simulink model "dc_motor_starter_design_v4"  (R2025a)
settings: Solver=VariableStepAuto  StartTime=0.0  StopTime=8  RelTol=1e-3
libraries: spsDiodeLib x8, spsCurrentMeasurementLib x6, spsMosfetLib x5, simulink x4, spsMeanLib x4, spsSeriesRLCBranchLib x4, spsVoltageMeasurementLib x3, spsDCVoltageSourceLib x2, eePwmGenerator x2, spsACVoltageSourceLib x1, spsDCMachineLib x1, spsFirstOrderFilterLib x1
settings Model: Creator=Lenovo  LastModifiedBy=kaand

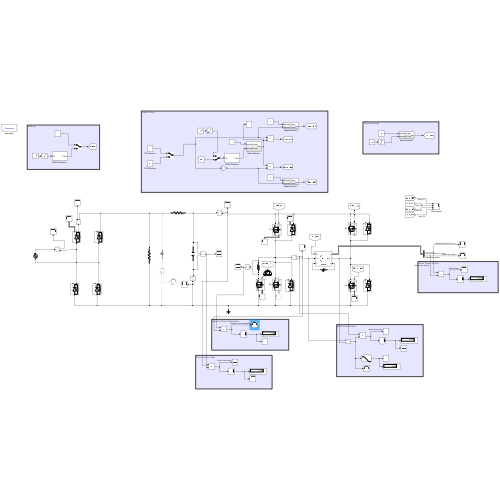
[thumbnail: Simulink's stored preview of the top-level diagram]
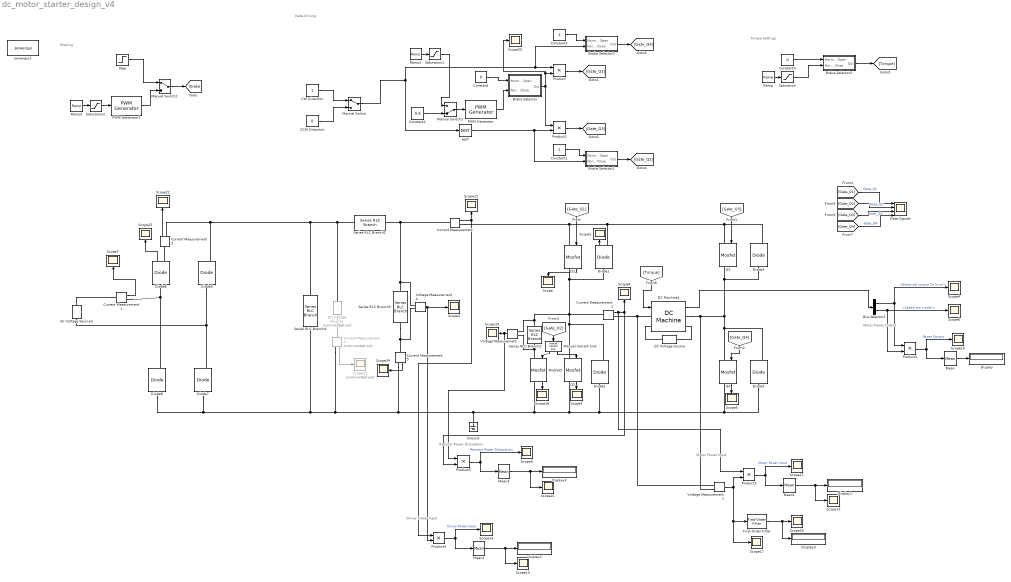
== system dc_motor_starter_design_v4 ==
  note: Torque Settings
  note: Gate Driving
  note: Resistor Power Dissipation
  note: Motor Power Input
  note: Motor Power Output
  note: Driver Power Input
  note: Braking
  AC Voltage Source3 : spsACVoltageSourceLib/AC Voltage Source  Amplitude=230  Phase=0  Frequency=50  SampleTime=0  Measurements=None  BusType=swing  Pref=10e3  Qref=0  Qmin=-inf  Qmax=+inf
  Brake Selector : Subsystem
  Brake Selector1 : Subsystem
  Brake Selector2 : Subsystem
  Brake Selector3 : Subsystem
  Bus Selector1 : BusSelector  OutputSignals=Electrical torque Te (n m),Speed wm (rad/s)
  CCW Direction : Constant  Value=0
  CW Direction : Constant
  Constant : Constant  Value=0
  Constant1 : Constant
  Constant2 : Constant  Value=0.6
  Constant3 : Constant
  Constant4 : Constant  Value=0
  Current Measurement{,1..3,5} (5 alike) : spsCurrentMeasurementLib/Current Measurement  PhasorSimulation=off  OutputType=Complex  PSBequivalent=0
  Current Measurement4 : spsCurrentMeasurementLib/Current Measurement  Commented=on  PhasorSimulation=off  OutputType=Complex  PSBequivalent=0
  DC Machine1 : spsDCMachineLib/DC Machine  PresetModel=No  MechanicalLoad=Torque TL  FieldType=Wound  ShowDetailedParameters=on  MeasurementBus=off  RLa="[ 0.8  0.0125]"  RLf="[ 210  23]"  Laf=1.8  MachineConstant=Torque constant (N.m/A)  Ke=1.8  Kt=1.8  J=1  Bm=0  Tf=0  w0=1  Ifinit=1.04761904756944  TsPowergui=0  TsBlock=-1
  DC Voltage Source : spsDCVoltageSourceLib/DC Voltage Source  Amplitude=220  Measurements=None
  DC Voltage Source1 : spsDCVoltageSourceLib/DC Voltage Source  Commented=on  Amplitude=200  Measurements=None
  Diode{1..8} (8 alike) : spsDiodeLib/Diode  Ron=0.036  Lon=0  Vf=1.1  IC=0  UseSnubber=0  Rs=500  Cs=250e-9  Measurements=on
  Display{,1..4} (5 alike) : Display
  First-Order Filter : spsFirstOrderFilterLib/First-Order Filter  FilterType=Lowpass  Tc=800e-6  Ts=0  Initialize=off  Vac_Init=[0, 0, 60]  Vdc_Init=0  PlotResponse=off  FreqRange="[0,  200,  1]"
  Gate Signals : Scope  NumInputPorts=4
      settings: ActiveDisplayYMinimum=-0.0065041846728933761  ActiveDisplayYMaximum=1.2434958153271063  DataLoggingVariableName=ScopeData21
  Ground : spsGroundLib/Ground  LConnTagsString=a
  Manual Variant Sink : simulink/Signal Routing/Manual Variant Sink  NumChoices=2  LabelModeActiveChoice=V_1
  Manual Switch : ManualSwitch
  Manual Switch1 : ManualSwitch  CurrentSetting=0
  Manual Switch2 : ManualSwitch
  Mean{,1..3} (4 alike) : spsMeanLib/Mean  Freq=50  Vinit=0  Ts=0
  Mosfet5 : spsMosfetLib/Mosfet  Ron=0.078  Lon=0  Rd=0.01  Vfd=0.7  IC=0  Rs=1e5  Cs=inf  Measurements=on
  NOT : Logic  Operator=NOT  IconShape=distinctive  AllPortsSameDT=off  OutDataTypeStr=boolean
  PWM Generator : eePwmGenerator/PWM Generator  CarrCount=Up  Tper=1/20e3  Tdelay=0  Ts=5e-6
  PWM Generator1 : eePwmGenerator/PWM Generator  CarrCount=Up  Tper=1/20e3  Tdelay=0  Ts=5e-6
  Product{,1..5} (6 alike) : Product
  Q{1..4} (4 alike) : spsMosfetLib/Mosfet  Ron=0.078  Lon=0  Rd=0.01  Vfd=0.7  IC=0  Rs=1e5  Cs=inf  Measurements=on
  Ramp : simulink/Sources/Ramp  slope=50  start=2  InitialOutput=0
  Ramp1 : simulink/Sources/Ramp  slope=0.2  start=0  InitialOutput=0
  Ramp2 : simulink/Sources/Ramp  slope=0.5  start=3.5  InitialOutput=0
  Saturation : Saturate  UpperLimit=20  LowerLimit=0
  Saturation1 : Saturate  UpperLimit=0.8  LowerLimit=0
  Saturation2 : Saturate  UpperLimit=1  LowerLimit=0
  Scope{,1..22,24..25} (25 alike) : Scope
      Scope settings: ActiveDisplayYMinimum=-11.583479260065536  ActiveDisplayYMaximum=104.1740277954152  DataLoggingVariableName=ScopeData2
      Scope1 settings: ActiveDisplayYMinimum=-28.46919774047009  ActiveDisplayYMaximum=256.22277966423093
      Scope10 settings: ActiveDisplayYMinimum=624.50186928798541  ActiveDisplayYMaximum=1429.223755324701  DataLoggingVariableName=ScopeData10
      Scope11 settings: ActiveDisplayYMinimum=-2401.1873049076858  ActiveDisplayYMaximum=10839.355284849147  DataLoggingVariableName=ScopeData12
      Scope12 settings: ActiveDisplayYMinimum=-11.566622282825097  ActiveDisplayYMaximum=104.03628291708009  DataLoggingVariableName=ScopeData11
      Scope13 settings: DataLoggingVariableName=ScopeData13
      Scope14 settings: ActiveDisplayYMinimum=762.41218453396561  ActiveDisplayYMaximum=2945.0127128560962  DataLoggingVariableName=ScopeData14
      Scope15 settings: DataLoggingVariableName=ScopeData15
      Scope16 settings: ActiveDisplayYMinimum=-15.282258817280159  ActiveDisplayYMaximum=137.54032935552146  DataLoggingVariableName=ScopeData16
      Scope17 settings: ActiveDisplayYMinimum=-36.761209497993441  ActiveDisplayYMaximum=226.2370362043749  DataLoggingVariableName=ScopeData17
      Scope18 settings: DataLoggingVariableName=ScopeData18
      Scope19 settings: ActiveDisplayYMinimum=-12.603657312689416  ActiveDisplayYMaximum=103.81128270332889  DataLoggingVariableName=ScopeData19
      Scope2 settings: ActiveDisplayYMinimum=-226.88562627237616  ActiveDisplayYMaximum=25.20951403026401  DataLoggingVariableName=ScopeData3
      Scope20 settings: ActiveDisplayYMinimum=-0.12499999999999997  ActiveDisplayYMaximum=1.125  DataLoggingVariableName=ScopeData20
      Scope21 settings: ActiveDisplayYMinimum=-1899.3717072203649  ActiveDisplayYMaximum=211.04566043540314  DataLoggingVariableName=ScopeData9
      Scope22 settings: ActiveDisplayYMinimum=-4.8702002164060625  ActiveDisplayYMaximum=43.751360629299874  DataLoggingVariableName=ScopeData23
      Scope24 settings: ActiveDisplayYMinimum=-110.97493026864629  ActiveDisplayYMaximum=197.18570910939735  DataLoggingVariableName=ScopeData25
      Scope25 settings: ActiveDisplayYMinimum=-19.273015293489355  ActiveDisplayYMaximum=173.45713764140422  DataLoggingVariableName=ScopeData26
      Scope3 settings: ActiveDisplayYMinimum=-122.00523332078208  ActiveDisplayYMaximum=132.92248346873072  DataLoggingVariableName=ScopeData4
      Scope4 settings: ActiveDisplayYMinimum=-65.687848106790781  ActiveDisplayYMaximum=243.58123391583604
      Scope5 settings: ActiveDisplayYMinimum=-1.20703950016334  ActiveDisplayYMaximum=7.0075960496809362  DataLoggingVariableName=ScopeData6
      Scope6 settings: ActiveDisplayYMinimum=-7.9782501074375674  ActiveDisplayYMaximum=71.8134310936752  DataLoggingVariableName=ScopeData5
      Scope7 settings: ActiveDisplayYMinimum=-170.79208981594385  ActiveDisplayYMaximum=171.40567773098573  DataLoggingVariableName=ScopeData7
      Scope8 settings: ActiveDisplayYMinimum=-136.4523697158933  ActiveDisplayYMaximum=140.46232304628771  DataLoggingVariableName=ScopeData8
      Scope9 settings: ActiveDisplayYMinimum=-2178.2019033970919  ActiveDisplayYMaximum=243.07898503401125  DataLoggingVariableName=ScopeData22
  Scope23 : Scope  Commented=on
      settings: ActiveDisplayYMinimum=-145.42462200714976  ActiveDisplayYMaximum=71.245138524934077  DataLoggingVariableName=ScopeData24
  Series RLC Branch1 : spsSeriesRLCBranchLib/Series RLC Branch  LConnTagsString=__new0  RConnTagsString=__new0  BranchType=R  Resistance=0.001  Inductance=1e-3  SetiL0=off  InitialCurrent=0  Capacitance=15000e-6  Setx0=off  InitialVoltage=0  Measurements=None
  Series RLC Branch2 : spsSeriesRLCBranchLib/Series RLC Branch  LConnTagsString=__new0  RConnTagsString=__new0  BranchType=R  Resistance=5  Inductance=1e-3  SetiL0=off  InitialCurrent=0  Capacitance=15000e-6  Setx0=off  InitialVoltage=0  Measurements=None
  Series RLC Branch3 : spsSeriesRLCBranchLib/Series RLC Branch  LConnTagsString=__new0  RConnTagsString=__new0  BranchType=C  Resistance=1  Inductance=1e-3  SetiL0=off  InitialCurrent=0  Capacitance=1500e-6  Setx0=off  InitialVoltage=0  Measurements=None
  Series RLC Branch4 : spsSeriesRLCBranchLib/Series RLC Branch  LConnTagsString=__new0  RConnTagsString=__new0  BranchType=R  Resistance=27e3  Inductance=1e-3  SetiL0=off  InitialCurrent=0  Capacitance=15000e-6  Setx0=off  InitialVoltage=0  Measurements=None
  Step : Step  Time=3.5  SampleTime=0
  Voltage Measurement : spsVoltageMeasurementLib/Voltage Measurement  PhasorSimulation=off  OutputType=Complex  PSBequivalent=0
  Voltage Measurement1 : spsVoltageMeasurementLib/Voltage Measurement  PhasorSimulation=off  OutputType=Complex  PSBequivalent=0
  Voltage Measurement2 : spsVoltageMeasurementLib/Voltage Measurement  PhasorSimulation=off  OutputType=Complex  PSBequivalent=0
  powergui2 : sps_lib/powergui  Priority=1  SimulationMode=Continuous  SampleTime=50e-6  frequency=60  Iterations=50  frequencyindice=0  Pbase=100e6  ErrMax=1e-4  UnitsV=kV  UnitsW=MW  buscounter=0  FunctionMessages=off  echomessages=off  EnableUseOfTLC=off  CurrentSourceSwitches=off  DisableSnubberDevices=off  DisableRonSwitches=off  DisableVfSwitches=off  DisplayEquations=off  AutomaticDiscreteSolvers=off  SolverType=Tustin/Backward Euler (TBE)  Interpol=off  ExternalGateDelay=off  methode=off  Ts=100  x0status=blocks  SPID=on  SwTol=0  HookPort=off  NonlinearTolerance=1e-4  nMaxIteration=100  ContinueOnMaxIteration=off  RestoreLinks=warning  ResistiveCurrentMeasurement=off  Frange=[0:2:500]  Ylog=off  Xlog=on  ShowGrid=off  save=off  variable=ZData  structure=0  ZoomFFT=off  StartTime=0.0  cycles=1  DisplayStyle=1  fundamental=60  FreqAxis=off  MaxFrequency=1000  frequencyindicesteady=1  RmsSteady=1  display=off
  tag scope: Brake=global
  wires:
  Current Measurement1/1 -> Scope7/1
  Voltage Measurement2/1 -> Scope1/1, Product4/2
  Current Measurement/1 -> Product4/1, Scope12/1
  CW Direction/1 -> Manual Switch/1
  CCW Direction/1 -> Manual Switch/2
  Manual Switch/1 -> NOT/1, Brake Selector2/2(Normally Close), Product/1
  NOT/1 -> Brake Selector1/2(Normally Close), Product1/2
  Bus Selector1/2 -> Scope6/1, Product2/2  "<Speed wm (rad/s)>"
  Bus Selector1/1 -> Product2/1, Scope4/1  "<Electrical torque Te (n m)>"
  DC Machine1/1 -> Bus Selector1/1
  Ramp1/1 -> Saturation1/1
  Constant2/1 -> Manual Switch1/2
  Saturation1/1 -> Manual Switch1/1
  Manual Switch1/1 -> PWM Generator/1
  Q1/1 -> Scope/1
  Diode1/1 -> Scope2/1
  Q2/1 -> Scope3/1
  Q4/1 -> Scope5/1
  Current Measurement2/1 -> Scope8/1, Product5/2, Product3/1
  Product2/1 -> Mean/1, Scope10/1  "Power Output"
  Mean/1 -> Display/1
  Mean1/1 -> Scope13/1, Display1/1
  Product3/1 -> Mean1/1, Scope11/1  "Motor Power Input"
  Voltage Measurement1/1 -> Scope17/1, First-Order Filter/1, Product3/2
  Product4/1 -> Mean2/1, Scope14/1  "Driver Power Input"
  Mean2/1 -> Scope15/1, Display2/1
  First-Order Filter/1 -> Display3/1, Scope16/1
  Mosfet5/1 -> Scope18/1
  Voltage Measurement/1 -> Product5/1, Scope19/1
  Brake Selector/1(Out) -> Product1/1, Scope20/1, Product/2
  Constant/1 -> Brake Selector/1(Normally Open)
  PWM Generator/1 -> Brake Selector/2(Normally Close)
  Product/1 -> [Gate_Q1]
  [Gate_Q1] -> Q1/1
  [Gate_Q3] -> Q3/1
  Product1/1 -> [Gate_Q3]
  [Gate_Q1] -> Gate Signals/1  "Gate_Q1"
  [Gate_Q2] -> Gate Signals/2  "Gate_Q2"
  [Gate_Q3] -> Gate Signals/3  "Gate_Q3"
  [Gate_Q4] -> Gate Signals/4  "Gate_Q4"
  Constant1/1 -> Brake Selector1/1(Normally Open)
  Brake Selector1/1(Out) -> [Gate_Q2]
  Constant3/1 -> Brake Selector2/1(Normally Open)
  Brake Selector2/1(Out) -> [Gate_Q4]
  [Gate_Q4] -> Q4/1
  Saturation2/1 -> PWM Generator1/1
  Manual Switch2/1 -> [Brake]
  Step/1 -> Manual Switch2/1
  PWM Generator1/1 -> Manual Switch2/2
  Ramp2/1 -> Saturation2/1
  Ramp/1 -> Saturation/1
  Saturation/1 -> Brake Selector3/2(Normally Close)
  Constant4/1 -> Brake Selector3/1(Normally Open)
  Brake Selector3/1(Out) -> [Torque]
  [Torque] -> DC Machine1/1
  [Gate_Q2] -> Manual Variant Sink/1
  Manual Variant Sink/1 -> Mosfet5/1
  Manual Variant Sink/2 -> Q2/1
  Product5/1 -> Mean3/1, Scope9/1  "Resistor Power Dissipation"
  Mean3/1 -> Scope21/1, Display4/1
  Current Measurement3/1 -> Scope22/1
  Current Measurement4/1 -> Scope23/1
  Current Measurement5/1 -> Scope24/1
  Diode6/1 -> Scope25/1
  connections:
  Diode7/RConn1 -- Diode5/LConn1 -- AC Voltage Source3/LConn1
  Diode6/LConn1 -- Diode8/RConn1 -- Current Measurement1/RConn1
  Q1/RConn1 -- Diode1/LConn1 -- Voltage Measurement/LConn1 -- Series RLC Branch2/LConn1 -- Q2/LConn1 -- Diode2/RConn1 -- Current Measurement2/LConn1
  AC Voltage Source3/RConn1 -- Current Measurement1/LConn1
  Diode1/RConn1 -- Diode3/RConn1 -- Q3/LConn1 -- Q1/LConn1 -- Current Measurement/RConn1
  Diode8/LConn1 -- Diode7/LConn1 -- Series RLC Branch4/RConn1 -- Mosfet5/RConn1 -- Q2/RConn1 -- Q4/RConn1 -- Diode4/LConn1 -- Diode2/LConn1 -- Ground/LConn1 -- Current Measurement5/RConn1 -- Current Measurement4/RConn1
  DC Voltage Source/LConn1 -- DC Machine1/RConn2
  DC Voltage Source/RConn1 -- DC Machine1/LConn2
  Diode5/RConn1 -- Current Measurement3/RConn1 -- Series RLC Branch4/LConn1 -- Series RLC Branch1/LConn1 -- DC Voltage Source1/RConn1
  Current Measurement2/RConn1 -- DC Machine1/LConn1 -- Voltage Measurement1/LConn1
  Q4/LConn1 -- Diode4/RConn1 -- DC Machine1/RConn1 -- Voltage Measurement1/LConn2 -- Diode3/LConn1 -- Q3/RConn1
  Current Measurement/LConn1 -- Series RLC Branch1/RConn1 -- Voltage Measurement2/LConn1 -- Series RLC Branch3/LConn1
  Mosfet5/LConn1 -- Voltage Measurement/LConn2 -- Series RLC Branch2/RConn1
  Diode6/RConn1 -- Current Measurement3/LConn1
  DC Voltage Source1/LConn1 -- Current Measurement4/LConn1
  Series RLC Branch3/RConn1 -- Current Measurement5/LConn1 -- Voltage Measurement2/LConn2

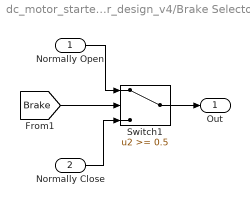
== system dc_motor_starter_design_v4/Brake Selector ==
  Normally Open : Inport
  Normally Close : Inport  Port=2
  Switch1 : Switch  Threshold=0.5  SaturateOnIntegerOverflow=off  InputSameDT=off
  Out : Outport
  wires:
  Normally Close/1 -> Switch1/3
  [Brake] -> Switch1/2
  Normally Open/1 -> Switch1/1
  Switch1/1 -> Out/1

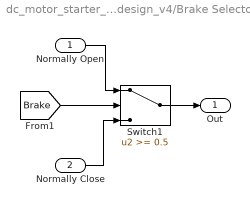
== system dc_motor_starter_design_v4/Brake Selector1 ==
  Normally Open : Inport
  Normally Close : Inport  Port=2
  Switch1 : Switch  Threshold=0.5  SaturateOnIntegerOverflow=off  InputSameDT=off
  Out : Outport
  wires:
  Normally Close/1 -> Switch1/3
  [Brake] -> Switch1/2
  Normally Open/1 -> Switch1/1
  Switch1/1 -> Out/1

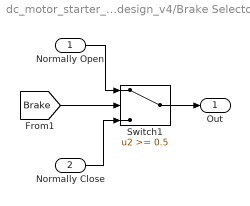
== system dc_motor_starter_design_v4/Brake Selector2 ==
  Normally Open : Inport
  Normally Close : Inport  Port=2
  Switch1 : Switch  Threshold=0.5  SaturateOnIntegerOverflow=off  InputSameDT=off
  Out : Outport
  wires:
  Normally Close/1 -> Switch1/3
  [Brake] -> Switch1/2
  Normally Open/1 -> Switch1/1
  Switch1/1 -> Out/1

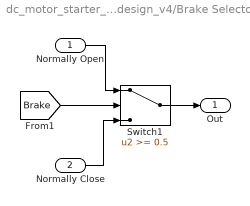
== system dc_motor_starter_design_v4/Brake Selector3 ==
  Normally Open : Inport
  Normally Close : Inport  Port=2
  Switch1 : Switch  Threshold=0.5  SaturateOnIntegerOverflow=off  InputSameDT=off
  Out : Outport
  wires:
  Normally Close/1 -> Switch1/3
  [Brake] -> Switch1/2
  Normally Open/1 -> Switch1/1
  Switch1/1 -> Out/1
